simulink library "ad9136"  (R2021a)
settings: Solver=VariableStepAuto  StartTime=0.0  StopTime=10.0  RelTol=1e-3
undefined symbols (not defined in the file): Fdata, Res, tessitura
settings Model: Creator=zhouxxxx  LastModifiedBy=zhouxxxx

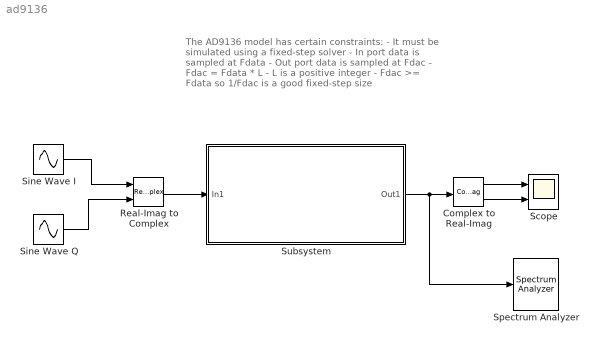
== system ad9136 ==
  note: The AD9136 model has  certain constraints:
      |   - It must be simulated using a fixed-step solver
      |   - In port data is sampled at Fdata
      |   - Out port data is sampled at Fdac
      |   - Fdac = Fdata * L
      |   - L is a positive integer
      |   - Fdac >= Fdata so 1/Fdac is a good fixed-step size
  Complex to Real-Imag : ComplexToRealImag
  Real-Imag to Complex : RealImagToComplex
  Scope : Scope  NumInputPorts=2
  Sine Wave I : Sin  SineType=Sample based  Amplitude=2^(Res-1)  Bias=2^(Res-1)  Frequency=2*pi*tessitura  Samples=Samples_per_period  SampleTime=1/Fdata
  Sine Wave Q : Sin  SineType=Sample based  Amplitude=2^(Res-1)  Bias=2^(Res-1)  Frequency=2*pi*tessitura  Phase=-pi/2  Samples=Samples_per_period  SampleTime=1/Fdata  Offset=N_offset_samples
  Spectrum Analyzer : SpectrumAnalyzer
  Subsystem : Subsystem  mask{L=1, InvSinc=Disabled, Fdata=Fdata}
      mask prompts: L "Interpolation:"; InvSinc "Inverse SINC"
      settings: OpenFcn=mylib2
      mask TypeOptions L: 1 | 2 | 4 | 8
      mask TypeOptions InvSinc: Disabled | Enabled
      mask Display: disp('AD9316')
  wires:
  Sine Wave I/1 -> Real-Imag to Complex/1
  Complex to Real-Imag/1 -> Scope/1
  Complex to Real-Imag/2 -> Scope/2
  Subsystem/1(Out1) -> Spectrum Analyzer/1, Complex to Real-Imag/1
  Real-Imag to Complex/1 -> Subsystem/1(In1)
  Sine Wave Q/1 -> Real-Imag to Complex/2

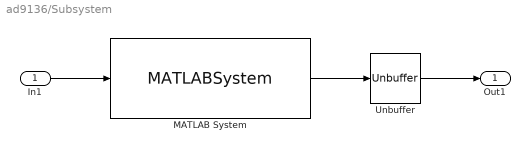
== system ad9136/Subsystem ==
  In1 : Inport
  MATLAB System : MATLABSystem  DialogController=sysobjdialog.BlockDynDialog  System=AD9136_sysobj  Interpolation=1  Fdata=Fdata  InvSinc=Disabled  OutputConfig=Normalized  SimulateUsing=Interpreted execution
      mask Type: AD9136_sysobj
      mask Display:
      | disp('AD9136');
      | port_label('input',1,'in (Code)');
      | port_label('output',1,'out (A)');
  Unbuffer : Unbuffer
  Out1 : Outport
  wires:
  In1/1 -> MATLAB System/1
  MATLAB System/1 -> Unbuffer/1
  Unbuffer/1 -> Out1/1
